simulink model "ErroSimulacao"  (R2020b)
settings: Solver=FixedStepDiscrete  StartTime=0.0  StopTime=20  FixedStep=1  RelTol=1e-3
InitFcn:
  | CarregaTabelas
  | Ts=10;
  | Freq=40;
  | PChegada=30;
  | VazaoIni=Interpola(Freq,PChegada*1.019716,MatrizSimulador,3)
undefined symbols (not defined in the file): Interpola, MatrizSimulador
settings Model: Creator=leize  LastModifiedBy=leize

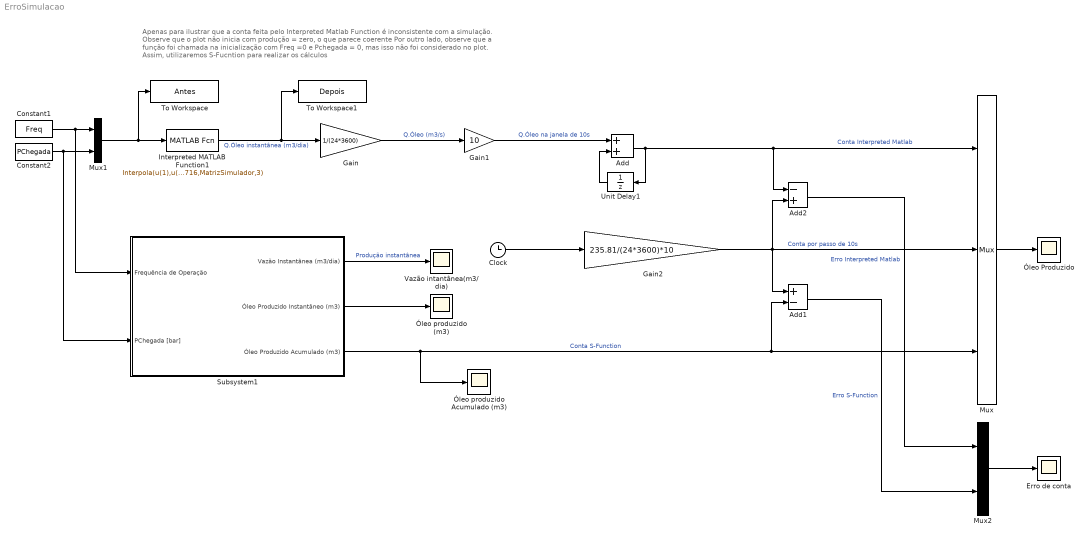
== system ErroSimulacao ==
  note: Apenas para ilustrar que a conta feita pelo Interpreted Matlab Function é inconsistente com a simulação.
      | Observe que o plot não inicia com produção = zero, o que parece coerente
      | Por outro lado, observe que a função foi chamada na inicialização com Freq =0 e Pchegada = 0, mas isso não foi considerado no plot. Assim, utilizaremos S-Fucntion para realizar os cálculos
  Add : Sum
  Add1 : Sum  Inputs=+-
  Add2 : Sum  Inputs=-+
  Clock : Clock
  Constant1 : Constant  Value=Freq
  Constant2 : Constant  Value=PChegada
  Erro de conta : Scope
  Gain : Gain  Gain=1/(24*3600)
  Gain1 : Gain  Gain=10
  Gain2 : Gain  Gain=235.81/(24*3600)*10
  Interpreted MATLAB Function1 : MATLABFcn  MATLABFcn=Interpola(u(1),u(2)*1.019716,MatrizSimulador,3)
  Mux : Mux  Inputs=3
  Mux1 : Mux  Inputs=2
  Mux2 : Mux  Inputs=2
  Subsystem1 : Subsystem  mask{MatrizSimulador=MatrizSimulador, DeltaT=Ts, QIni=VazaoIni}
      mask prompts: MatrizSimulador "Matriz do Simulador Petrobras"; DeltaT "Periodo de amostragem (s)"; QIni "Vazao Inicial (m3/dia)"
  To Workspace : ToWorkspace  VariableName=Antes  SaveFormat=Timeseries  SampleTime=-1
  To Workspace1 : ToWorkspace  VariableName=Depois  SaveFormat=Timeseries  SampleTime=-1
  Unit Delay1 : UnitDelay  SampleTime=-1  HasFrameUpgradeWarning=on
  Vazão intantânea(m3/dia) : Scope
  Óleo Produzido : Scope
  Óleo produzido (m3) : Scope
  Óleo produzido Acumulado (m3) : Scope
  wires:
  Unit Delay1/1 -> Add/2
  Gain1/1 -> Add/1  "Q.Óleo na janela de 10s"
  Mux1/1 -> To Workspace/1, Interpreted MATLAB Function1/1
  Gain/1 -> Gain1/1  "Q.Óleo (m3/s)"
  Interpreted MATLAB Function1/1 -> To Workspace1/1, Gain/1  "Q.Óleo instantânea (m3/dia)"
  Constant1/1 -> Subsystem1/1(Frequência de Operação), Mux1/1
  Constant2/1 -> Subsystem1/2(PChegada [bar]), Mux1/2
  Clock/1 -> Gain2/1
  Add/1 -> Add2/1, Mux/1, Unit Delay1/1  "Conta Interpreted Matlab"
  Mux/1 -> Óleo Produzido/1
  Subsystem1/3(Óleo Produzido Acumulado (m3)) -> Óleo produzido Acumulado (m3)/1, Add1/2, Mux/3  "Conta S-Function"
  Subsystem1/2("Óleo Produzido Instantâneo (m3) ") -> Óleo produzido (m3)/1
  Subsystem1/1(Vazão Instantânea (m3/dia)) -> Vazão intantânea(m3/dia)/1  "Produção instantânea"
  Gain2/1 -> Add2/2, Add1/1, Mux/2  "Conta por passo de 10s"
  Add2/1 -> Mux2/1  "Erro Interpreted Matlab"
  Add1/1 -> Mux2/2  "Erro S-Function"
  Mux2/1 -> Erro de conta/1

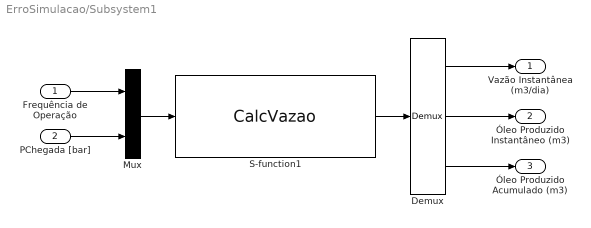
== system ErroSimulacao/Subsystem1 ==
  Frequência de Operação : Inport
  PChegada [bar] : Inport  Port=2
  Demux : Demux  Outputs=3
  Mux : Mux  Inputs=2
  S-function1 : S-Function  FunctionName=CalcVazao  Parameters=MatrizSimulador,DeltaT,QIni  SFunctionDeploymentMode=off  EnableBusSupport=off
  Vazão Instantânea (m3/dia) : Outport
  "Óleo Produzido Instantâneo (m3) " : Outport  Port=2
  Óleo Produzido Acumulado (m3) : Outport  Port=3
  wires:
  PChegada [bar]/1 -> Mux/2
  Frequência de Operação/1 -> Mux/1
  Mux/1 -> S-function1/1
  S-function1/1 -> Demux/1
  Demux/2 -> "Óleo Produzido Instantâneo (m3) "/1
  Demux/3 -> Óleo Produzido Acumulado (m3)/1
  Demux/1 -> Vazão Instantânea (m3/dia)/1
